simulink model "Robot"  (R2015b)
settings: Solver=FixedStepAuto  StartTime=0.0  StopTime=10.0  FixedStep=0.1  RelTol=1e-3
settings Model: Creator=Deepak  LastModifiedBy=Deepak

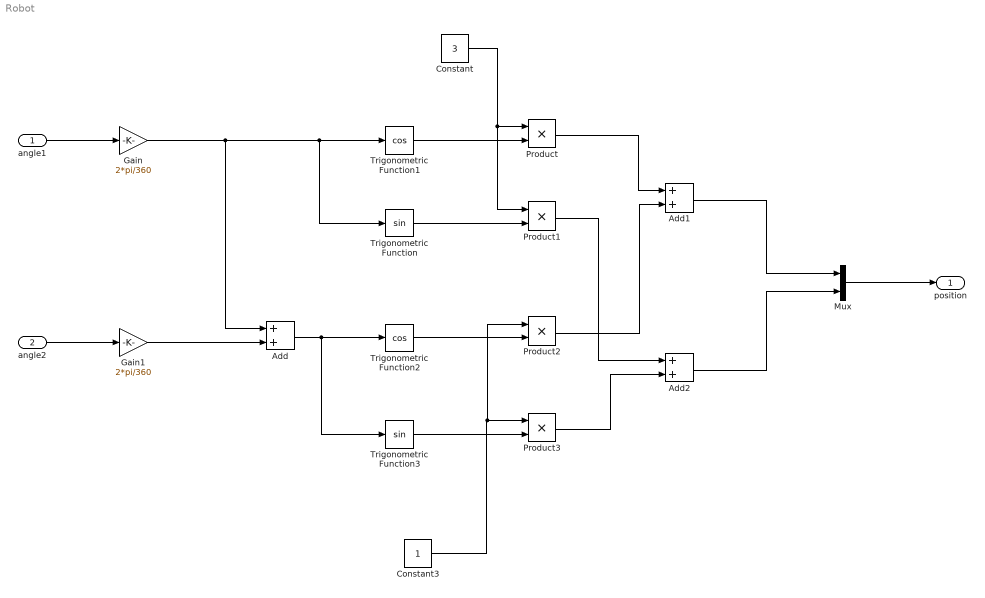
== system Robot ==
  angle1 : Inport
      settings: AttributesFormatString=angle
  angle2 : Inport  Port=2
      settings: AttributesFormatString=angle
  Add : Sum
  Add1 : Sum
  Add2 : Sum
  Constant : Constant  Value=3
  Constant3 : Constant
  Gain : Gain  Gain=2*pi/360
  Gain1 : Gain  Gain=2*pi/360
  Mux : Mux  Inputs=2
  Product{,1..3} (4 alike) : Product
  Trigonometric Function : Trigonometry
  Trigonometric Function1 : Trigonometry  Operator=cos
  Trigonometric Function2 : Trigonometry  Operator=cos
  Trigonometric Function3 : Trigonometry
  position : Outport
  wires:
  Mux/1 -> position/1
  angle1/1 -> Gain/1
  angle2/1 -> Gain1/1
  Gain/1 -> Add/1, Trigonometric Function/1, Trigonometric Function1/1
  Gain1/1 -> Add/2
  Add/1 -> Trigonometric Function3/1, Trigonometric Function2/1
  Trigonometric Function1/1 -> Product/2
  Trigonometric Function2/1 -> Product2/2
  Product/1 -> Add1/1
  Product2/1 -> Add1/2
  Constant/1 -> Product1/1, Product/1
  Trigonometric Function/1 -> Product1/2
  Constant3/1 -> Product2/1, Product3/1
  Trigonometric Function3/1 -> Product3/2
  Product1/1 -> Add2/1
  Product3/1 -> Add2/2
  Add1/1 -> Mux/1
  Add2/1 -> Mux/2
